simulink model "controllo_spazio_degli_stati"  (R2019b)
settings: Solver=VariableStepAuto  StartTime=0.0  StopTime=10.0  MaxStep=1e-3  RelTol=1e-3
undefined symbols (not defined in the file or in its folder): Ao, Bo, Co, DiscIntNeverNeededParam, H, K, L, Ts
libraries: cstblocks x1
settings Model: Creator=jacobi  LastModifiedBy=manue

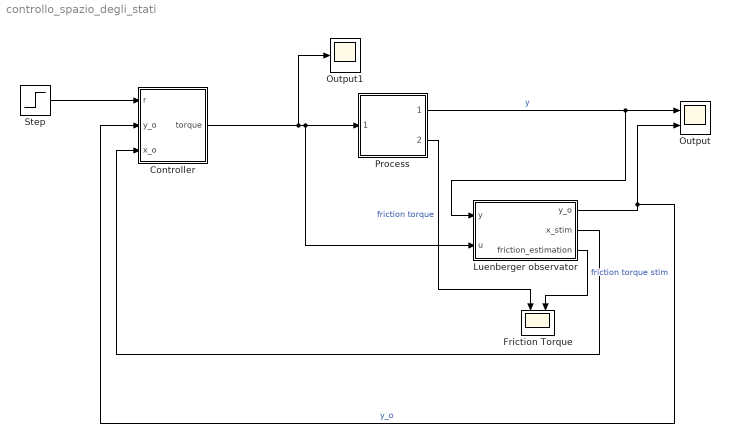
== system controllo_spazio_degli_stati ==
  Controller : Subsystem
  Friction Torque : Scope  NumInputPorts=2
  Luenberger observator : Subsystem
  Output : Scope  NumInputPorts=2
  Output1 : Scope
  Process : Subsystem
  Step : Step  Time=4  SampleTime=0
  wires:
  Luenberger observator/1(y_o) -> Output/2, Controller/2(y_o)  "y_o"
  Process/1(Position) -> Luenberger observator/1(y), Output/1  "y"
  Process/2(Friction torque) -> Friction Torque/1  "friction torque"
  Luenberger observator/3(friction_estimation) -> Friction Torque/2  "friction torque stim"
  Controller/1(torque) -> Output1/1, Luenberger observator/2(u), Process/1(Torque)
  Step/1 -> Controller/1(r)
  Luenberger observator/2(x_stim) -> Controller/3(x_o)

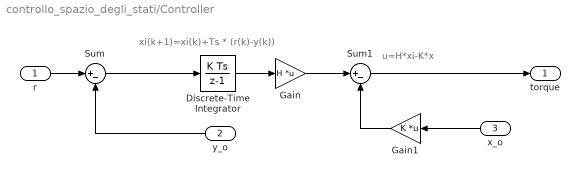
== system controllo_spazio_degli_stati/Controller ==
  note: u=H*xi-K*x
  note: xi(k+1)=xi(k)+Ts * (r(k)-y(k))
  r : Inport
  y_o : Inport  Port=2
  x_o : Inport  Port=3
  Discrete-Time Integrator : DiscreteIntegrator  gainval=1  SampleTime=Ts  ICPrevOutput=DiscIntNeverNeededParam  ICPrevScaledInput=DiscIntNeverNeededParam
  Gain : Gain  Gain=H  Multiplication=Matrix(K*u)
  Gain1 : Gain  Gain=K  Multiplication=Matrix(K*u)
  Sum : Sum  Inputs=|+-
  Sum1 : Sum  Inputs=|+-
  torque : Outport
  wires:
  Sum1/1 -> torque/1
  Discrete-Time Integrator/1 -> Gain/1
  x_o/1 -> Gain1/1
  Gain/1 -> Sum1/1
  r/1 -> Sum/1
  y_o/1 -> Sum/2
  Gain1/1 -> Sum1/2
  Sum/1 -> Discrete-Time Integrator/1

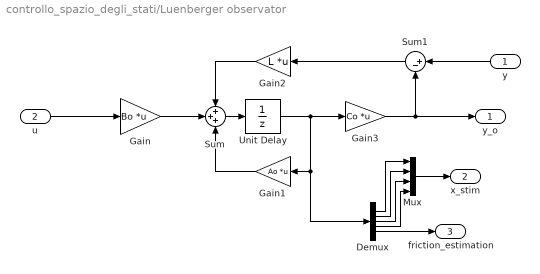
== system controllo_spazio_degli_stati/Luenberger observator ==
  y : Inport
  u : Inport  Port=2
  Demux : Demux  Outputs=5
  Gain : Gain  Gain=Bo  Multiplication=Matrix(K*u)
  Gain1 : Gain  Gain=Ao  Multiplication=Matrix(K*u)
  Gain2 : Gain  Gain=L  Multiplication=Matrix(K*u)
  Gain3 : Gain  Gain=Co  Multiplication=Matrix(K*u)
  Mux : Mux
  Sum : Sum  Inputs=+++
  Sum1 : Sum  Inputs=|+-
  Unit Delay : UnitDelay  SampleTime=Ts  HasFrameUpgradeWarning=on
  y_o : Outport
  x_stim : Outport  Port=2
  friction_estimation : Outport  Port=3
  wires:
  Unit Delay/1 -> Gain3/1, Demux/1, Gain1/1
  Sum/1 -> Unit Delay/1
  Gain1/1 -> Sum/3
  Gain/1 -> Sum/2
  Gain3/1 -> Sum1/2, y_o/1
  Sum1/1 -> Gain2/1
  Gain2/1 -> Sum/1
  u/1 -> Gain/1
  y/1 -> Sum1/1
  Demux/5 -> friction_estimation/1
  Demux/4 -> Mux/4
  Demux/3 -> Mux/3
  Demux/2 -> Mux/2
  Demux/1 -> Mux/1
  Mux/1 -> x_stim/1

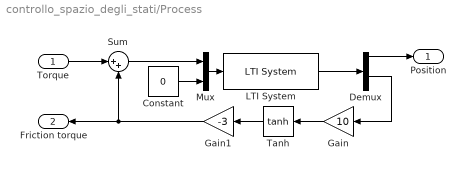
== system controllo_spazio_degli_stati/Process ==
  Torque : Inport
  Constant : Constant  Value=0
  Demux : Demux
  Gain : Gain  Gain=10
  Gain1 : Gain  Gain=-3
  LTI System : cstblocks/LTI System  sys=model  IC=[]
  Mux : Mux  Inputs=2
  Sum : Sum  Inputs=|++
  Tanh : Trigonometry  Operator=tanh
  Position : Outport
  Friction torque : Outport  Port=2
  wires:
  Sum/1 -> Mux/1
  Torque/1 -> Sum/1
  LTI System/1 -> Demux/1
  Demux/1 -> Position/1
  Demux/3 -> Gain/1
  Tanh/1 -> Gain1/1
  Gain/1 -> Tanh/1
  Gain1/1 -> Friction torque/1, Sum/2
  Mux/1 -> LTI System/1
  Constant/1 -> Mux/2
